simulink model "ped_s6_spwm"  (R2023b)
settings: Solver=VariableStepAuto  StartTime=0.0  StopTime=10.0  RelTol=1e-3
libraries: spsMosfetLib x4, spsDCVoltageSourceLib x1, spsRMSLib x1, spsSawtoothGeneratorLib x1, spsSeriesRLCBranchLib x1, spsVoltageMeasurementLib x1, sps_lib x1
settings Model: Creator=JAYRAJ  LastModifiedBy=JAYRAJ

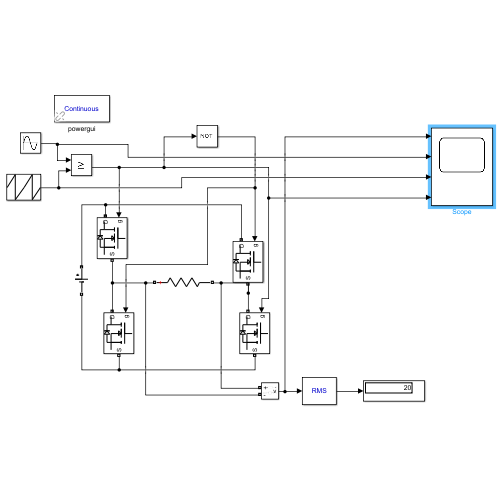
[thumbnail: Simulink's stored preview of the top-level diagram]
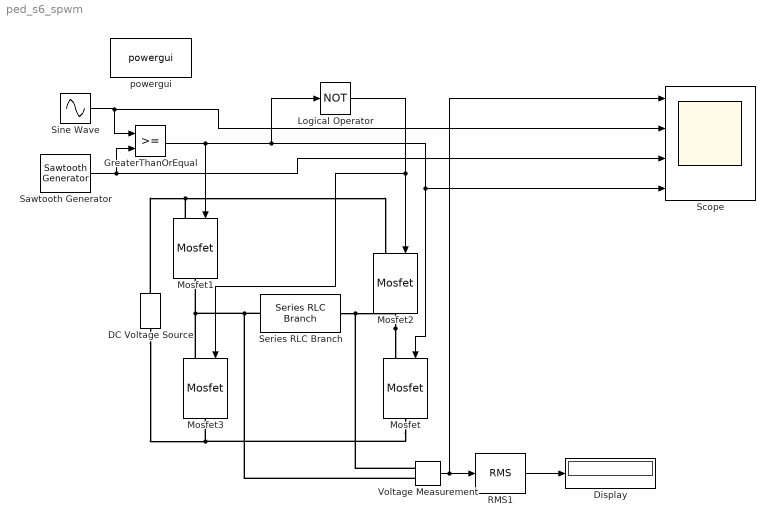
== system ped_s6_spwm ==
  DC Voltage Source : spsDCVoltageSourceLib/DC Voltage Source  Amplitude=24  Measurements=None
  Display : Display
  GreaterThanOrEqual : RelationalOperator  OutDataTypeStr=boolean  RndMeth=Simplest  InputSameDT=off
  Logical Operator : Logic  Operator=NOT  AllPortsSameDT=off  OutDataTypeStr=boolean
  Mosfet{,1..3} (4 alike) : spsMosfetLib/Mosfet  Ron=0.1  Lon=0  Rd=0.01  Vfd=0  IC=0  Rs=1e5  Cs=inf  Measurements=off
  RMS1 : spsRMSLib/RMS  TrueRMS=on  Freq=50  RMSInit=120  Ts=0
  Sawtooth Generator : spsSawtoothGeneratorLib/Sawtooth Generator  Freq=1e3  Phase=180  Ts=0
  Scope : Scope  NumInputPorts=4
  Series RLC Branch : spsSeriesRLCBranchLib/Series RLC Branch  LConnTagsString=__new0  RConnTagsString=__new0  BranchType=R  Resistance=1  Inductance=1e-3  SetiL0=off  InitialCurrent=0  Capacitance=1e-6  Setx0=off  InitialVoltage=0  Measurements=None
  Sine Wave : Sin  Frequency=314  SampleTime=0
  Voltage Measurement : spsVoltageMeasurementLib/Voltage Measurement  PhasorSimulation=off  OutputType=Complex  PSBequivalent=0
  powergui : sps_lib/powergui  Priority=1  SimulationMode=Continuous  SampleTime=50e-6  frequency=60  Iterations=50  frequencyindice=0  Pbase=100e6  ErrMax=1e-4  UnitsV=kV  UnitsW=MW  buscounter=0  FunctionMessages=off  echomessages=off  EnableUseOfTLC=off  CurrentSourceSwitches=off  DisableSnubberDevices=off  DisableRonSwitches=off  DisableVfSwitches=off  DisplayEquations=off  AutomaticDiscreteSolvers=off  SolverType=Tustin/Backward Euler (TBE)  Interpol=off  ExternalGateDelay=off  methode=off  Ts=100  x0status=blocks  SPID=on  SwTol=0  HookPort=off  NonlinearTolerance=1e-4  nMaxIteration=100  ContinueOnMaxIteration=off  RestoreLinks=warning  ResistiveCurrentMeasurement=off  Frange=[0:2:500]  Ylog=off  Xlog=on  ShowGrid=off  save=off  variable=ZData  structure=0  ZoomFFT=off  StartTime=0.0  cycles=1  DisplayStyle=1  fundamental=60  FreqAxis=off  MaxFrequency=1000  frequencyindicesteady=1  RmsSteady=1  display=off
  wires:
  RMS1/1 -> Display/1
  Voltage Measurement/1 -> RMS1/1, Scope/1
  Sine Wave/1 -> Scope/2, GreaterThanOrEqual/1
  Sawtooth Generator/1 -> GreaterThanOrEqual/2, Scope/3
  GreaterThanOrEqual/1 -> Mosfet/1, Scope/4, Logical Operator/1, Mosfet1/1
  Logical Operator/1 -> Mosfet2/1, Mosfet3/1
  connections:
  Mosfet3/LConn1 -- Series RLC Branch/LConn1 -- Voltage Measurement/LConn2 -- Mosfet1/RConn1
  Mosfet2/RConn1 -- Voltage Measurement/LConn1 -- Series RLC Branch/RConn1 -- Mosfet/LConn1
  Mosfet/RConn1 -- DC Voltage Source/LConn1 -- Mosfet3/RConn1
  DC Voltage Source/RConn1 -- Mosfet2/LConn1 -- Mosfet1/LConn1
